simulink model "schiewerwurf"  (R2016b)
settings: Solver=VariableStepAuto  StartTime=0.0  StopTime=10.0  RelTol=1e-3
values from neighbouring files (symbols this model uses):
  g = -9.81    [schieferwurf_param.m]
  h = 5    [schieferwurf_param.m]
  vx0 = 10    [schieferwurf_param.m]
  vz0 = 10    [schieferwurf_param.m]
libraries: simulink x1
settings Model: Creator=local  LastModifiedBy=local

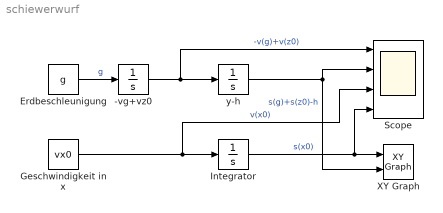
== system schiewerwurf ==
  -vg+vz0 : Integrator  InitialCondition=vz0
  Erdbeschleunigung : Constant  Value=g
  Geschwindigkeit in x : Constant  Value=vx0
  Integrator : Integrator
  Scope : Scope  NumInputPorts=4
  XY Graph : simulink/Sinks/XY Graph  xmin=0  xmax=30  ymin=0  ymax=15  st=-1
  y-h : Integrator  InitialCondition=h
  wires:
  Erdbeschleunigung/1 -> -vg+vz0/1  "g"
  Integrator/1 -> XY Graph/1, Scope/4  "s(x0)"
  -vg+vz0/1 -> y-h/1, Scope/1  "-v(g)+v(z0)"
  Geschwindigkeit in x/1 -> Scope/3, Integrator/1  "v(x0)"
  y-h/1 -> Scope/2, XY Graph/2  "s(g)+s(z0)-h"
